simulink model "Simulink_asserv_Disc_5mars"  (R2024a)
settings: Solver=VariableStepAuto  StartTime=0.0  StopTime=1000  FixedStep=0.01  RelTol=1e-3
model workspace (MAT data in the model file):
  AmbiantTemp = 25
  CondSig_mesureTemp_Gain = 4.35
  CondSig_mesureTemp_Vsub = 1.95
  DivTen_mesureTemp_R_pullup = 10000
  DivTen_mesureTemp_Vcc = 5
  Estimateur_alpha = 0.5
  Filtre_mesureTemp_deno = [0.0033 1]
  Gain_Comparateur_VoltageControle = 0.32
  RC_deno = [3.22e-08 3.04e-05 0.00955 1]
  SourceCourant_Gain_Vcontrole_vers_A = 3.1564
  ThermoRes_SHTEMP_A = 0.003354
  ThermoRes_SHTEMP_B = 0.00026
  ThermoRes_SHTEMP_C = 1.6e-06
  ThermoRes_SHTEMP_D = 6.3e-08
  ThermoRes_SH_A = -14.65719
  ThermoRes_SH_B = 4798.842
  ThermoRes_SH_C = -115334
  ThermoRes_SH_D = -3730535
  ThermoRes_SH_R_nom = 10000
libraries: simulink x3
settings Model: SimulationMode=rapid-accelerator  Creator=alcot161  LastModifiedBy=ALCOT161

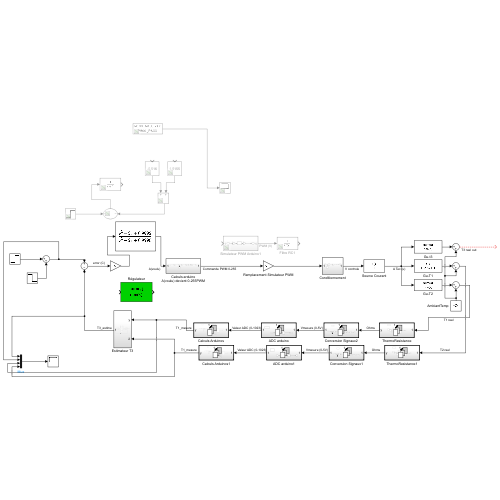
[thumbnail: Simulink's stored preview of the top-level diagram]
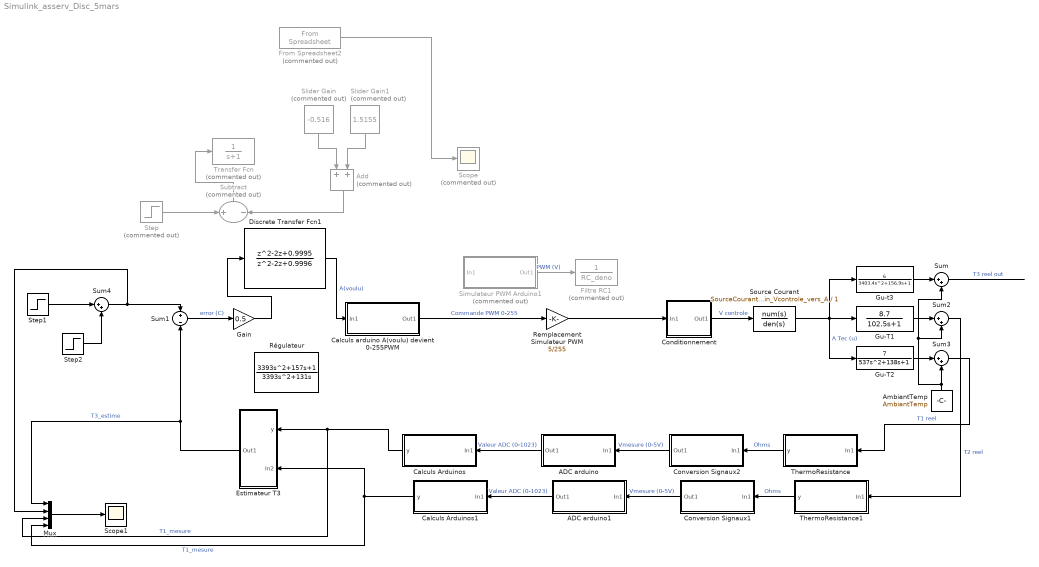
== system Simulink_asserv_Disc_5mars ==
  ADC arduino : Subsystem  TreatAsAtomicUnit=on
  ADC arduino1 : Subsystem  TreatAsAtomicUnit=on
  Add : Sum  Commented=on
  AmbiantTemp : Constant  Value=AmbiantTemp
  Calculs Arduinos : Subsystem  TreatAsAtomicUnit=on
  Calculs Arduinos1 : Subsystem  TreatAsAtomicUnit=on
  Calculs arduino A(voulu) devient 0-255PWM : Subsystem
  Conditionnement : Subsystem
  Conversion Signaux1 : Subsystem  TreatAsAtomicUnit=on
  Conversion Signaux2 : Subsystem  TreatAsAtomicUnit=on
  Discrete Transfer Fcn1 : DiscreteTransferFcn  Numerator=[1 -2 0.9995]  Denominator=[1 -2 0.9996]
  Estimateur T3 : Subsystem
  Filtre RC1 : TransferFcn  Commented=on  Denominator=RC_deno
  From Spreadsheet2 : FromSpreadsheet  Commented=on  FileName=N600_N800.xlsx  SheetName=P600_P800  Range=A2:A100  SampleTime=-1
  Gain : Gain  Gain=0.5
  Gu-T1 : TransferFcn  Numerator=[8.7]  Denominator=[102.5 1]
  Gu-T2 : TransferFcn  Numerator=[7]  Denominator=[537 138 1]
  Gu-t3 : TransferFcn  Numerator=[6]  Denominator=[3403.4 156.9 1]
  Mux : Mux
  Remplacement Simulateur PWM : Gain  Gain=5/255
  Régulateur : TransferFcn  Numerator=[3393 157 1]  Denominator=[3393 131 0]
  Scope : Scope  Commented=on
  Scope1 : Scope
  Simulateur PWM Arduino1 : Subsystem  Commented=on
  Slider Gain : simulink/Math Operations/Slider Gain  Commented=on  gain=-0.516  low=-2  high=2
  Slider Gain1 : simulink/Math Operations/Slider Gain  Commented=on  gain=1.5155  low=-2  high=2
  Source Courant : TransferFcn  Numerator=SourceCourant_Gain_Vcontrole_vers_A  Denominator=1
  Step : Step  Commented=on  SampleTime=0
  Step1 : Step  Time=10  Before=25  After=27  SampleTime=0.05
  Step2 : Step  Time=500  After=-4  SampleTime=0.05
  Subtract : Sum  Commented=on  Inputs=+-
  Sum{,2..4} (4 alike) : Sum  Inputs=|++
  Sum1 : Sum  Inputs=+|-  SampleTime=0
  ThermoResistance : Subsystem  TreatAsAtomicUnit=on
  ThermoResistance1 : Subsystem  TreatAsAtomicUnit=on
  Transfer Fcn : TransferFcn  Commented=on  Denominator=[1 1]
  wires:
  From Spreadsheet2/1 -> Scope/1
  Subtract/1 -> Transfer Fcn/1
  Slider Gain/1 -> Add/1
  Slider Gain1/1 -> Add/2
  Add/1 -> Subtract/2
  Step/1 -> Subtract/1
  Sum1/1 -> Gain/1  "error (C)"
  Calculs arduino A(voulu) devient 0-255PWM/1(Out1) -> Remplacement Simulateur PWM/1  "Commande PWM 0-255"
  Remplacement Simulateur PWM/1 -> Conditionnement/1(In1)
  Conditionnement/1(Out1) -> Source Courant/1  "V controle"
  Source Courant/1 -> Gu-T2/1, Gu-T1/1, Gu-t3/1  "A Tec (u)"
  Gu-t3/1 -> Sum/1
  Gu-T1/1 -> Sum2/1
  Gu-T2/1 -> Sum3/1
  AmbiantTemp/1 -> Sum/2, Sum2/2, Sum3/2
  Sum2/1 -> ThermoResistance1/1(In1)  "T2 reel"
  Sum3/1 -> ThermoResistance/1(In1)  "T1 reel"
  ThermoResistance/1(y) -> Conversion Signaux2/1(In1)  "Ohms"
  Conversion Signaux2/1(Out1) -> ADC arduino/1(In1)  "Vmesure (0-5V)"
  ADC arduino/1(Out1) -> Calculs Arduinos/1(In1)  "Valeur ADC (0-1023)"
  Calculs Arduinos/1(y) -> Mux/3, Estimateur T3/1(y)  "T1_mesure"
  Estimateur T3/1(Out1) -> Mux/1, Sum1/2  "T3_estime"
  Simulateur PWM Arduino1/1(Out1) -> Filtre RC1/1  "PWM (V)"
  Sum/1 -> ?  "T3 reel out"
  Gain/1 -> Discrete Transfer Fcn1/1
  Discrete Transfer Fcn1/1 -> Calculs arduino A(voulu) devient 0-255PWM/1(In1)  "A(voulu)"
  Step1/1 -> Sum4/1
  Step2/1 -> Sum4/2
  Mux/1 -> Scope1/1
  Sum4/1 -> Mux/2, Sum1/1
  Calculs Arduinos1/1(y) -> Estimateur T3/2(In2), Mux/4  "T1_mesure"
  ThermoResistance1/1(y) -> Conversion Signaux1/1(In1)  "Ohms"
  ADC arduino1/1(Out1) -> Calculs Arduinos1/1(In1)  "Valeur ADC (0-1023)"
  Conversion Signaux1/1(Out1) -> ADC arduino1/1(In1)  "Vmesure (0-5V)"

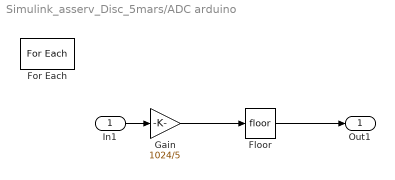
== system Simulink_asserv_Disc_5mars/ADC arduino ==
  In1 : Inport  Partition=on  PartitionDimension=1  PartitionWidth=1  PartitionOffset=0
  Floor : Rounding
  For Each : ForEach  DisableCoverage=on
  Gain : Gain  Gain=1024/5
  Out1 : Outport  ConcatenationDimension=1
  wires:
  In1/1 -> Gain/1
  Gain/1 -> Floor/1
  Floor/1 -> Out1/1

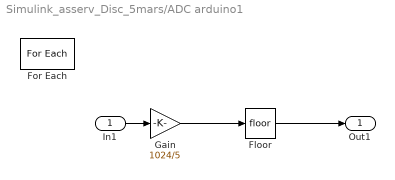
== system Simulink_asserv_Disc_5mars/ADC arduino1 ==
  In1 : Inport  Partition=on  PartitionDimension=1  PartitionWidth=1  PartitionOffset=0
  Floor : Rounding
  For Each : ForEach  DisableCoverage=on
  Gain : Gain  Gain=1024/5
  Out1 : Outport  ConcatenationDimension=1
  wires:
  In1/1 -> Gain/1
  Gain/1 -> Floor/1
  Floor/1 -> Out1/1

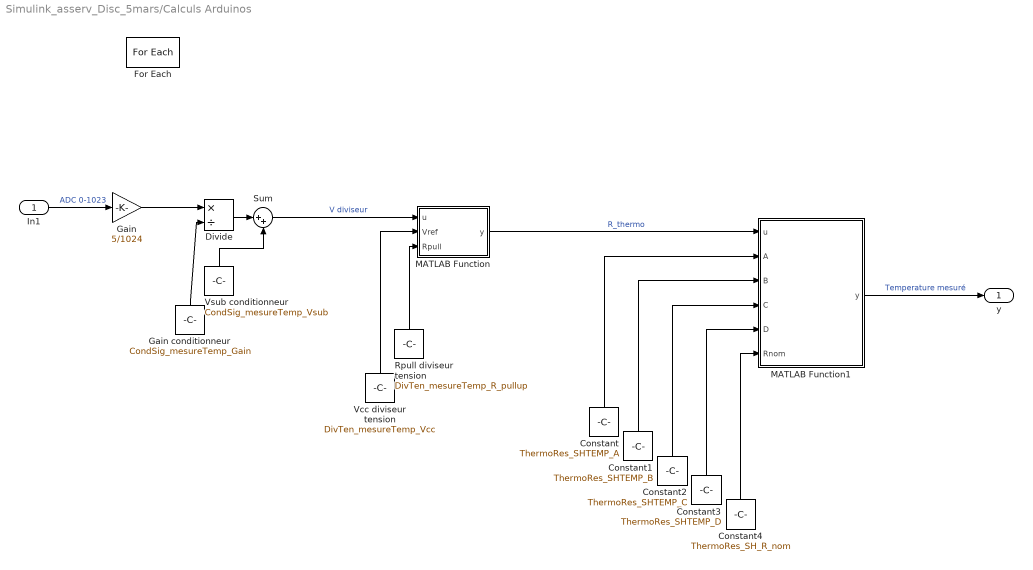
== system Simulink_asserv_Disc_5mars/Calculs Arduinos ==
  In1 : Inport  Partition=on  PartitionDimension=1  PartitionWidth=1  PartitionOffset=0
  Constant : Constant  Value=ThermoRes_SHTEMP_A
  Constant1 : Constant  Value=ThermoRes_SHTEMP_B
  Constant2 : Constant  Value=ThermoRes_SHTEMP_C
  Constant3 : Constant  Value=ThermoRes_SHTEMP_D
  Constant4 : Constant  Value=ThermoRes_SH_R_nom
  Divide : Product  Inputs=*/
  For Each : ForEach  DisableCoverage=on
  Gain : Gain  Gain=5/1024
  Gain conditionneur : Constant  Value=CondSig_mesureTemp_Gain
  MATLAB Function : MATLAB Function  TreatAsAtomicUnit=on
  MATLAB Function1 : MATLAB Function  TreatAsAtomicUnit=on
  Rpull diviseur tension : Constant  Value=DivTen_mesureTemp_R_pullup
  Sum : Sum  Inputs=|++
  Vcc diviseur tension : Constant  Value=DivTen_mesureTemp_Vcc
  Vsub conditionneur : Constant  Value=CondSig_mesureTemp_Vsub
  y : Outport  ConcatenationDimension=1
  wires:
  In1/1 -> Gain/1  "ADC 0-1023"
  Gain/1 -> Divide/1
  Gain conditionneur/1 -> Divide/2
  Divide/1 -> Sum/1
  Vsub conditionneur/1 -> Sum/2
  Sum/1 -> MATLAB Function/1(u)  "V diviseur"
  Rpull diviseur tension/1 -> MATLAB Function/3(Rpull)
  Vcc diviseur tension/1 -> MATLAB Function/2(Vref)
  MATLAB Function/1(y) -> MATLAB Function1/1(u)  "R_thermo"
  Constant/1 -> MATLAB Function1/2(A)
  Constant1/1 -> MATLAB Function1/3(B)
  Constant2/1 -> MATLAB Function1/4(C)
  Constant3/1 -> MATLAB Function1/5(D)
  Constant4/1 -> MATLAB Function1/6(Rnom)
  MATLAB Function1/1(y) -> y/1  "Temperature mesuré"

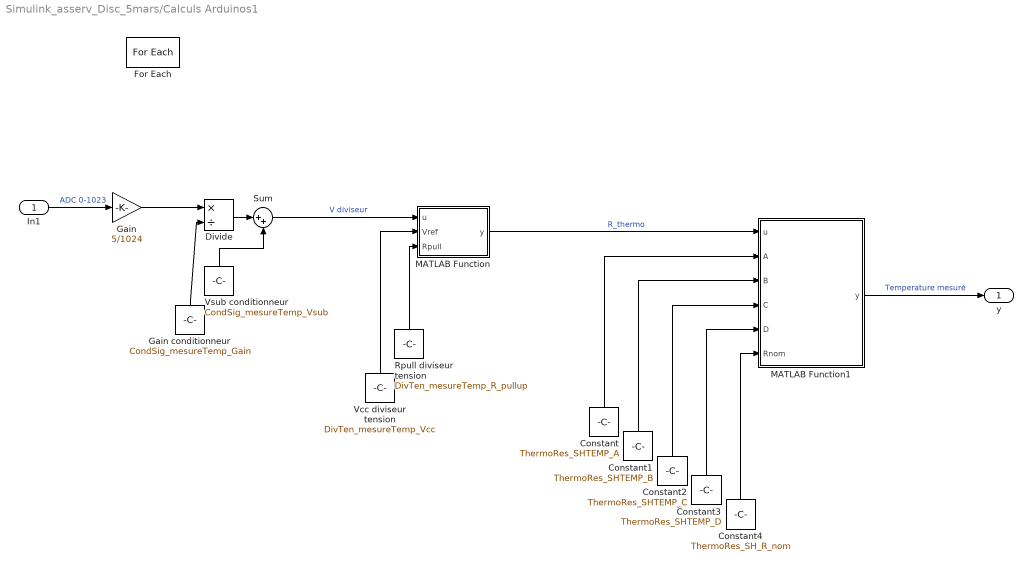
== system Simulink_asserv_Disc_5mars/Calculs Arduinos1 ==
  In1 : Inport  Partition=on  PartitionDimension=1  PartitionWidth=1  PartitionOffset=0
  Constant : Constant  Value=ThermoRes_SHTEMP_A
  Constant1 : Constant  Value=ThermoRes_SHTEMP_B
  Constant2 : Constant  Value=ThermoRes_SHTEMP_C
  Constant3 : Constant  Value=ThermoRes_SHTEMP_D
  Constant4 : Constant  Value=ThermoRes_SH_R_nom
  Divide : Product  Inputs=*/
  For Each : ForEach  DisableCoverage=on
  Gain : Gain  Gain=5/1024
  Gain conditionneur : Constant  Value=CondSig_mesureTemp_Gain
  MATLAB Function : MATLAB Function  TreatAsAtomicUnit=on
  MATLAB Function1 : MATLAB Function  TreatAsAtomicUnit=on
  Rpull diviseur tension : Constant  Value=DivTen_mesureTemp_R_pullup
  Sum : Sum  Inputs=|++
  Vcc diviseur tension : Constant  Value=DivTen_mesureTemp_Vcc
  Vsub conditionneur : Constant  Value=CondSig_mesureTemp_Vsub
  y : Outport  ConcatenationDimension=1
  wires:
  In1/1 -> Gain/1  "ADC 0-1023"
  Gain/1 -> Divide/1
  Gain conditionneur/1 -> Divide/2
  Divide/1 -> Sum/1
  Vsub conditionneur/1 -> Sum/2
  Sum/1 -> MATLAB Function/1(u)  "V diviseur"
  Rpull diviseur tension/1 -> MATLAB Function/3(Rpull)
  Vcc diviseur tension/1 -> MATLAB Function/2(Vref)
  MATLAB Function/1(y) -> MATLAB Function1/1(u)  "R_thermo"
  Constant/1 -> MATLAB Function1/2(A)
  Constant1/1 -> MATLAB Function1/3(B)
  Constant2/1 -> MATLAB Function1/4(C)
  Constant3/1 -> MATLAB Function1/5(D)
  Constant4/1 -> MATLAB Function1/6(Rnom)
  MATLAB Function1/1(y) -> y/1  "Temperature mesuré"

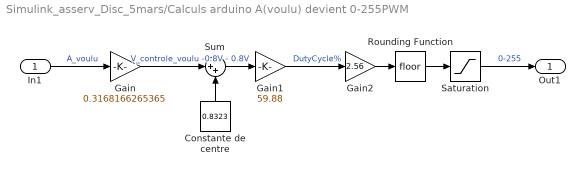
== system Simulink_asserv_Disc_5mars/Calculs arduino A(voulu) devient 0-255PWM ==
  In1 : Inport
  Constante de centre : Constant  Value=0.8323
  Gain : Gain  Gain=0.3168166265365
  Gain1 : Gain  Gain=59.88
  Gain2 : Gain  Gain=2.56  ParamMin=0  ParamMax=255.9  OutMin=[0]  OutMax=[255]
  Rounding Function : Rounding
  Saturation : Saturate  UpperLimit=255  LowerLimit=0  LinearizeAsGain=off
  Sum : Sum  Inputs=|++
  Out1 : Outport
  wires:
  In1/1 -> Gain/1  "A_voulu"
  Gain/1 -> Sum/1  "V_controle_voulu -0.8V - 0.8V"
  Sum/1 -> Gain1/1
  Constante de centre/1 -> Sum/2
  Gain1/1 -> Gain2/1  "DutyCycle%"
  Gain2/1 -> Rounding Function/1
  Rounding Function/1 -> Saturation/1
  Saturation/1 -> Out1/1  "0-255"

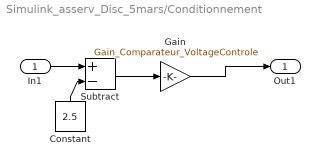
== system Simulink_asserv_Disc_5mars/Conditionnement ==
  In1 : Inport
  Constant : Constant  Value=2.5
  Gain : Gain  Gain=Gain_Comparateur_VoltageControle
  Subtract : Sum  Inputs=+-
  Out1 : Outport
  wires:
  In1/1 -> Subtract/1
  Constant/1 -> Subtract/2
  Subtract/1 -> Gain/1
  Gain/1 -> Out1/1

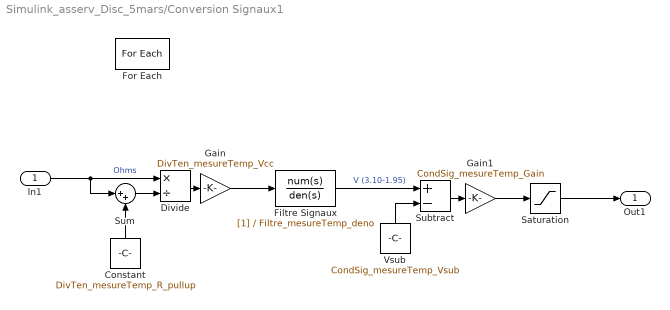
== system Simulink_asserv_Disc_5mars/Conversion Signaux1 ==
  In1 : Inport  Partition=on  PartitionDimension=1  PartitionWidth=1  PartitionOffset=0
  Constant : Constant  Value=DivTen_mesureTemp_R_pullup
  Divide : Product  Inputs=*/
  Filtre Signaux : TransferFcn  Denominator=Filtre_mesureTemp_deno
  For Each : ForEach  DisableCoverage=on
  Gain : Gain  Gain=DivTen_mesureTemp_Vcc
  Gain1 : Gain  Gain=CondSig_mesureTemp_Gain
  Saturation : Saturate  UpperLimit=5  LowerLimit=0
  Subtract : Sum  Inputs=+-
  Sum : Sum  Inputs=|++
  Vsub : Constant  Value=CondSig_mesureTemp_Vsub
  Out1 : Outport  ConcatenationDimension=1
  wires:
  In1/1 -> Sum/1, Divide/1  "Ohms"
  Sum/1 -> Divide/2
  Constant/1 -> Sum/2
  Divide/1 -> Gain/1
  Gain/1 -> Filtre Signaux/1
  Vsub/1 -> Subtract/2
  Filtre Signaux/1 -> Subtract/1  "V (3.10-1.95)"
  Subtract/1 -> Gain1/1
  Gain1/1 -> Saturation/1
  Saturation/1 -> Out1/1

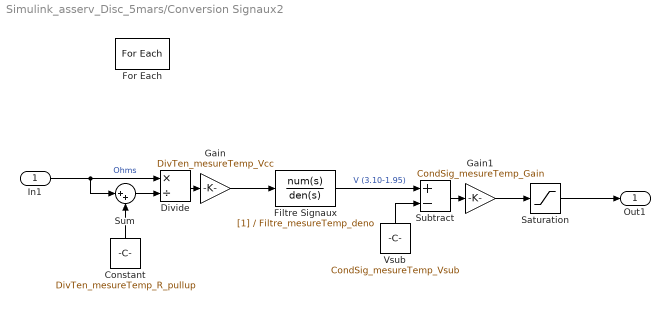
== system Simulink_asserv_Disc_5mars/Conversion Signaux2 ==
  In1 : Inport  Partition=on  PartitionDimension=1  PartitionWidth=1  PartitionOffset=0
  Constant : Constant  Value=DivTen_mesureTemp_R_pullup
  Divide : Product  Inputs=*/
  Filtre Signaux : TransferFcn  Denominator=Filtre_mesureTemp_deno
  For Each : ForEach  DisableCoverage=on
  Gain : Gain  Gain=DivTen_mesureTemp_Vcc
  Gain1 : Gain  Gain=CondSig_mesureTemp_Gain
  Saturation : Saturate  UpperLimit=5  LowerLimit=0
  Subtract : Sum  Inputs=+-
  Sum : Sum  Inputs=|++
  Vsub : Constant  Value=CondSig_mesureTemp_Vsub
  Out1 : Outport  ConcatenationDimension=1
  wires:
  In1/1 -> Sum/1, Divide/1  "Ohms"
  Sum/1 -> Divide/2
  Constant/1 -> Sum/2
  Divide/1 -> Gain/1
  Gain/1 -> Filtre Signaux/1
  Vsub/1 -> Subtract/2
  Filtre Signaux/1 -> Subtract/1  "V (3.10-1.95)"
  Subtract/1 -> Gain1/1
  Gain1/1 -> Saturation/1
  Saturation/1 -> Out1/1

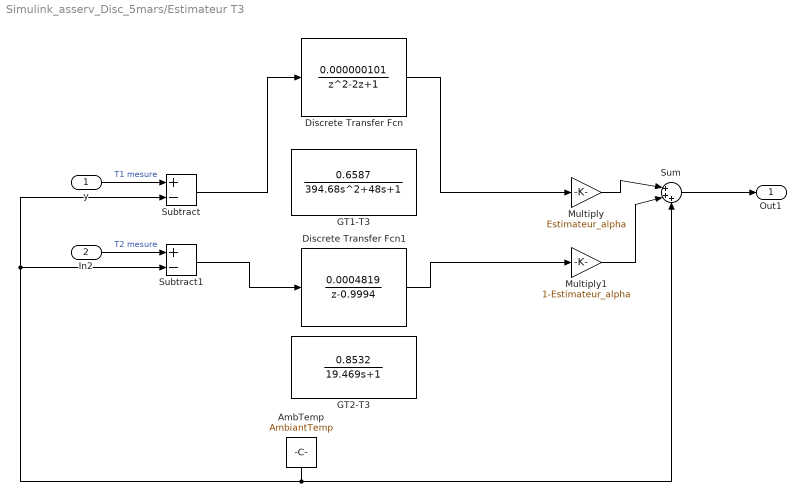
== system Simulink_asserv_Disc_5mars/Estimateur T3 ==
  y : Inport
  In2 : Inport  Port=2
  AmbTemp : Constant  Value=AmbiantTemp
  Discrete Transfer Fcn : DiscreteTransferFcn  Numerator=[0.000000101]  Denominator=[1 -2 1]
  Discrete Transfer Fcn1 : DiscreteTransferFcn  Numerator=[0.0004819]  Denominator=[1 -0.9994]
  GT1-T3 : TransferFcn  Numerator=[0.6587]  Denominator=[394.68 48 1]
  GT2-T3 : TransferFcn  Numerator=[0.8532]  Denominator=[19.469 1]
  Multiply : Gain  Gain=Estimateur_alpha
  Multiply1 : Gain  Gain=1-Estimateur_alpha
  Subtract : Sum  Inputs=+-
  Subtract1 : Sum  Inputs=+-
  Sum : Sum  Inputs=|+++
  Out1 : Outport
  wires:
  In2/1 -> Subtract1/1  "T2 mesure"
  Multiply/1 -> Sum/1
  Multiply1/1 -> Sum/2
  y/1 -> Subtract/1  "T1 mesure"
  Subtract/1 -> Discrete Transfer Fcn/1
  Subtract1/1 -> Discrete Transfer Fcn1/1
  Sum/1 -> Out1/1
  AmbTemp/1 -> Sum/3, Subtract1/2, Subtract/2
  Discrete Transfer Fcn/1 -> Multiply/1
  Discrete Transfer Fcn1/1 -> Multiply1/1

== system Simulink_asserv_Disc_5mars/Simulateur PWM Arduino1 ==
  In1 : Inport
  Gain1 : Gain  Gain=1/255
  Gain2 : Gain  Gain=5
  PWM : simulink/Discontinuities/PWM  DisableCoverage=on  Period=0.00204  InitialDelay=0  DisallowZeroDutyCycle=off  RunAtFixedTimeIntervals=off  SampleTime=0.1
  Out1 : Outport
  wires:
  Gain1/1 -> PWM/1
  PWM/1 -> Gain2/1
  In1/1 -> Gain1/1
  Gain2/1 -> Out1/1

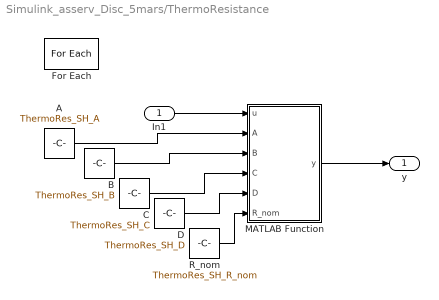
== system Simulink_asserv_Disc_5mars/ThermoResistance ==
  In1 : Inport  Partition=on  PartitionDimension=1  PartitionWidth=1  PartitionOffset=0
  A : Constant  Value=ThermoRes_SH_A
  B : Constant  Value=ThermoRes_SH_B
  C : Constant  Value=ThermoRes_SH_C
  D : Constant  Value=ThermoRes_SH_D
  For Each : ForEach  DisableCoverage=on
  MATLAB Function : MATLAB Function  TreatAsAtomicUnit=on
  R_nom : Constant  Value=ThermoRes_SH_R_nom
  y : Outport  ConcatenationDimension=1
  wires:
  In1/1 -> MATLAB Function/1(u)
  MATLAB Function/1(y) -> y/1
  A/1 -> MATLAB Function/2(A)
  B/1 -> MATLAB Function/3(B)
  C/1 -> MATLAB Function/4(C)
  D/1 -> MATLAB Function/5(D)
  R_nom/1 -> MATLAB Function/6(R_nom)

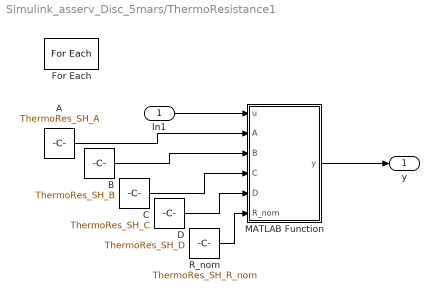
== system Simulink_asserv_Disc_5mars/ThermoResistance1 ==
  In1 : Inport  Partition=on  PartitionDimension=1  PartitionWidth=1  PartitionOffset=0
  A : Constant  Value=ThermoRes_SH_A
  B : Constant  Value=ThermoRes_SH_B
  C : Constant  Value=ThermoRes_SH_C
  D : Constant  Value=ThermoRes_SH_D
  For Each : ForEach  DisableCoverage=on
  MATLAB Function : MATLAB Function  TreatAsAtomicUnit=on
  R_nom : Constant  Value=ThermoRes_SH_R_nom
  y : Outport  ConcatenationDimension=1
  wires:
  In1/1 -> MATLAB Function/1(u)
  MATLAB Function/1(y) -> y/1
  A/1 -> MATLAB Function/2(A)
  B/1 -> MATLAB Function/3(B)
  C/1 -> MATLAB Function/4(C)
  D/1 -> MATLAB Function/5(D)
  R_nom/1 -> MATLAB Function/6(R_nom)

== matlab function Simulink_asserv_Disc_5mars/Calculs Arduinos1/MATLAB Function ==
  data: u input; y output; Vref input; Rpull input
function y = fcn(u, Vref, Rpull)

y = Rpull * (u/(Vref-u));

== matlab function Simulink_asserv_Disc_5mars/ThermoResistance/MATLAB Function ==
  data: u input; y output; A input; B input; C input; D input; R_nom input
function y = fcn(u, A, B, C, D, R_nom)
   
y = R_nom * exp(A + (B/(u+273.15)) + (C/((u + 273.15)^2)) + (D/((u + 273.15)^3)));

== matlab function Simulink_asserv_Disc_5mars/Calculs Arduinos/MATLAB Function ==
  data: u input; y output; Vref input; Rpull input
function y = fcn(u, Vref, Rpull)

y = Rpull * (u/(Vref-u));

== matlab function Simulink_asserv_Disc_5mars/Calculs Arduinos/MATLAB Function1 ==
  data: u input; y output; A input; B input; C input; D input; Rnom input
function y = fcn(u, A, B, C, D, Rnom)
    invT = A + B*log(u/Rnom) + C*(log(u/Rnom))^2 + D*(log(u/Rnom))^3;
    T = (1/invT) - 273.15;
y = T;

== matlab function Simulink_asserv_Disc_5mars/Calculs Arduinos1/MATLAB Function1 ==
  data: u input; y output; A input; B input; C input; D input; Rnom input
function y = fcn(u, A, B, C, D, Rnom)
    invT = A + B*log(u/Rnom) + C*(log(u/Rnom))^2 + D*(log(u/Rnom))^3;
    T = (1/invT) - 273.15;
y = T;

== matlab function Simulink_asserv_Disc_5mars/ThermoResistance1/MATLAB Function ==
  data: u input; y output; A input; B input; C input; D input; R_nom input
function y = fcn(u, A, B, C, D, R_nom)
   
y = R_nom * exp(A + (B/(u+273.15)) + (C/((u + 273.15)^2)) + (D/((u + 273.15)^3)));
